simulink model "sampleModel1463"  (R2023a)
settings: Solver=VariableStepAuto  StartTime=0.0  StopTime=10.0  RelTol=1e-3
libraries: hdlsllib x2, simulink x1
settings Model: Creator=user1  LastModifiedBy=user1

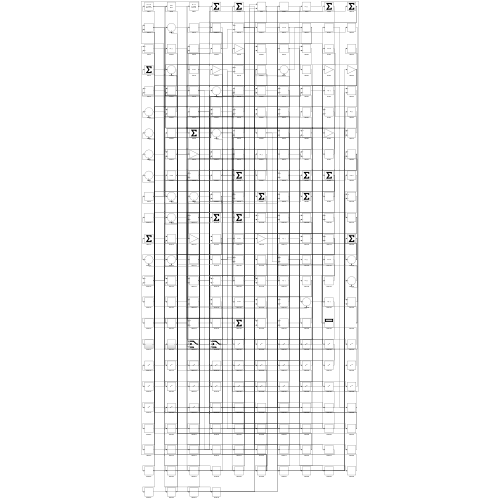
[thumbnail: Simulink's stored preview of the top-level diagram]
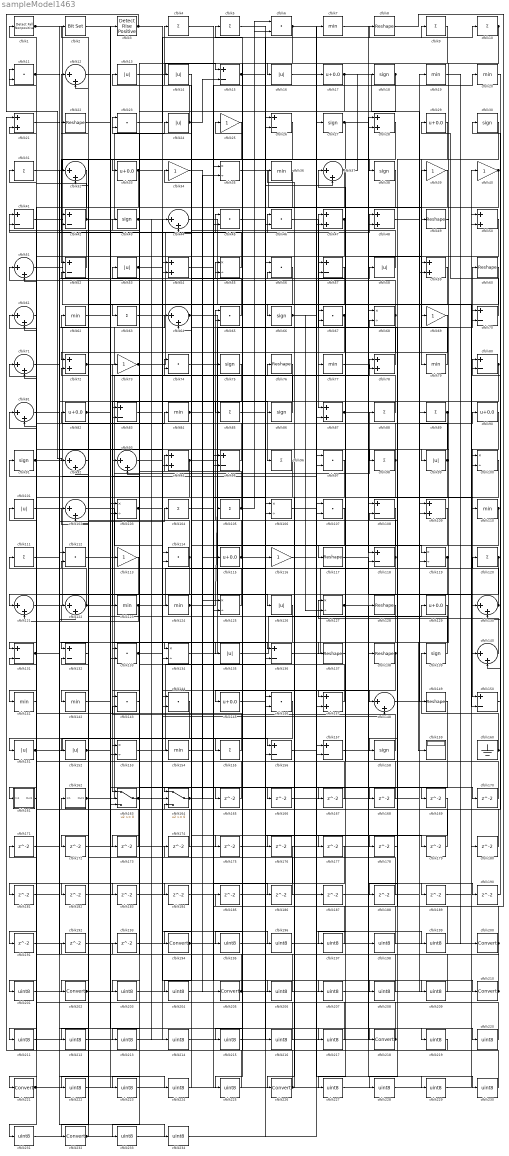
== system sampleModel1463 ==
  cfblk1 : hdlsllib/Logic and Bit Operations/Detect Fall Nonpositive  vinit=0  OutDataTypeStr=boolean
  cfblk{4..5,9..10,31,63,85,88..89,96,98,104..105,111,120,155} (16 alike) : Sum  Inputs=+
  cfblk{35,55,68,100,103,106,119,125,127,134,153} (11 alike) : Product  Inputs=*/  RndMeth=Zero  SaturateOnIntegerOverflow=on
  cfblk{13..14,16,24,53,58,99,101,126,135,151..152} (12 alike) : Abs  SaturateOnIntegerOverflow=off
  cfblk{12,32,37,44,51,61,64,71,81,92..93,102,121..122,130,140,148} (17 alike) : Sum  Inputs=|++
  cfblk{6,11,23,45..46,56,65,67,74,97,107,112,114,133,143..144,146} (17 alike) : DotProduct  OutDataTypeStr=Inherit: Inherit via internal rule
  cfblk{15,26,41..42,52,57,70,80,83,95,108,118,131..132,136,150,156..157} (18 alike) : Sum  Inputs=+-
  cfblk{21,28,47..48,50,54,59,72,78,87,94,109,147} (13 alike) : Sum
  cfblk{7,19..20,36,62,77,79,84,110,123..124,141..142,154} (14 alike) : MinMax
  cfblk{25,34,39..40,69,73,113,116} (8 alike) : Gain
  cfblk{17,29,33,82,90,115,129,145} (8 alike) : Bias  Bias=0.0  SaturateOnIntegerOverflow=off
  cfblk{8,22,49,60,76,117,128,137..138,149} (10 alike) : Reshape
  cfblk{18,27,30,38,43,66,75,86,91,139,158} (11 alike) : Signum
  cfblk159 : Display
  cfblk160 : Ground
  cfblk161 : Subsystem
      settings: LibrarySourceBlock=|
      | hdlsllib/Ports &
      | Subsystems/Subsystem
  cfblk162 : Subsystem
      settings: LibrarySourceBlock=|
      | hdlsllib/Ports &
      | Subsystems/Subsystem
  cfblk163 : Switch  SaturateOnIntegerOverflow=off  InputSameDT=off
  cfblk164 : Switch  SaturateOnIntegerOverflow=off  InputSameDT=off
  cfblk{165..193} (29 alike) : Delay  SampleTime=1
  cfblk{194,200,202,205,210,218,221,226,232} (9 alike) : DataTypeConversion  SaturateOnIntegerOverflow=off  RndMeth=Floor
  cfblk{195..199,201,203..204,206..209,211..217,219..220,222..225,227..231,233..234} (32 alike) : DataTypeConversion  OutDataTypeStr=uint8  SaturateOnIntegerOverflow=off  RndMeth=Floor
  cfblk2 : simulink/Logic and Bit Operations/Bit Set  iBit=0
      settings: LibrarySourceBlock=|
      | hdlsllib/Logic and Bit
      | Operations/Bit Set
  cfblk3 : hdlsllib/Logic and Bit Operations/Detect Rise Positive  vinit=0  OutDataTypeStr=boolean
  wires:
  cfblk58/1 -> cfblk23/1
  cfblk162/1(Out1) -> cfblk88/1, cfblk42/2
  cfblk122/1 -> cfblk76/1, cfblk112/2, cfblk61/2
  cfblk91/1 -> cfblk84/1, cfblk48/1
  cfblk114/1 -> cfblk62/1, cfblk141/1, cfblk121/1
  cfblk76/1 -> cfblk163/1
  cfblk115/1 -> cfblk65/1, cfblk209/1
  cfblk160/1 -> cfblk139/1, cfblk80/1
  cfblk138/1 -> cfblk165/1, cfblk166/1
  cfblk112/1 -> cfblk78/1
  cfblk152/1 -> cfblk55/2, cfblk219/1
  cfblk94/1 -> cfblk47/1, cfblk153/2, cfblk231/1
  cfblk1/1 -> cfblk118/1, cfblk94/2
  cfblk49/1 -> cfblk159/1
  cfblk107/1 -> cfblk194/1
  cfblk121/1 -> cfblk46/1
  cfblk70/1 -> cfblk29/1
  cfblk29/1 -> cfblk79/1
  cfblk79/1 -> cfblk39/1
  cfblk22/1 -> cfblk155/1
  cfblk87/1 -> cfblk147/1, cfblk110/1
  cfblk109/1 -> cfblk117/1
  cfblk128/1 -> cfblk133/1
  cfblk63/1 -> cfblk66/1
  cfblk134/1 -> cfblk60/1
  cfblk3/1 -> cfblk92/1, cfblk196/1
  cfblk45/1 -> cfblk8/1
  cfblk18/1 -> cfblk85/1, cfblk195/1
  cfblk151/1 -> cfblk156/1, cfblk55/1, cfblk131/2
  cfblk64/1 -> cfblk119/1, cfblk186/1
  cfblk62/1 -> cfblk3/1
  cfblk95/1 -> cfblk83/1
  cfblk126/1 -> cfblk143/1
  cfblk24/1 -> cfblk4/1, cfblk15/2
  cfblk98/1 -> cfblk57/2, cfblk175/1
  cfblk6/1 -> cfblk16/1, cfblk230/1
  cfblk90/1 -> cfblk150/1
  cfblk161/1(Out1) -> cfblk11/1
  cfblk74/1 -> cfblk126/1
  cfblk43/1 -> cfblk164/2, cfblk208/1
  cfblk9/1 -> cfblk145/1
  cfblk129/1 -> cfblk134/1
  cfblk44/1 -> cfblk87/1
  cfblk40/1 -> cfblk92/2, cfblk158/1, cfblk44/2
  cfblk99/1 -> cfblk113/1, cfblk72/2, cfblk61/1
  cfblk56/1 -> cfblk63/1
  cfblk135/1 -> cfblk129/1
  cfblk139/1 -> cfblk91/1
  cfblk20/1 -> cfblk162/1(In1)
  cfblk17/1 -> cfblk149/1, cfblk153/1
  cfblk27/1 -> cfblk70/2, cfblk167/1
  cfblk78/1 -> cfblk13/1
  cfblk19/1 -> cfblk200/1
  cfblk31/1 -> cfblk38/1
  cfblk35/1 -> cfblk49/1
  cfblk146/1 -> cfblk232/1
  cfblk13/1 -> cfblk15/1
  cfblk46/1 -> cfblk77/1
  cfblk15/1 -> cfblk119/2, cfblk6/1, cfblk69/1, cfblk178/1
  cfblk37/1 -> cfblk133/2, cfblk18/1
  cfblk21/1 -> cfblk218/1
  cfblk150/1 -> cfblk30/1
  cfblk60/1 -> cfblk72/1
  cfblk97/1 -> cfblk202/1
  cfblk88/1 -> cfblk53/1
  cfblk104/1 -> cfblk75/1
  cfblk33/1 -> cfblk114/2, cfblk163/3
  cfblk118/1 -> cfblk132/1, cfblk94/1
  cfblk148/1 -> cfblk90/1
  cfblk72/1 -> cfblk7/1, cfblk58/1
  cfblk32/1 -> cfblk131/1
  cfblk110/1 -> cfblk136/2, cfblk225/1
  cfblk53/1 -> cfblk134/2, cfblk148/1
  cfblk55/1 -> cfblk41/1
  cfblk54/1 -> cfblk210/1
  cfblk153/1 -> cfblk116/1
  cfblk123/1 -> cfblk46/2, cfblk121/2
  cfblk141/1 -> cfblk31/1
  cfblk136/1 -> cfblk68/1
  cfblk68/1 -> cfblk51/1, cfblk102/2
  cfblk131/1 -> cfblk104/1, cfblk136/1
  cfblk84/1 -> cfblk95/2, cfblk64/2, cfblk20/1
  cfblk52/1 -> cfblk12/1
  cfblk80/1 -> cfblk96/1, cfblk144/2, cfblk228/1
  cfblk106/1 -> cfblk10/1
  cfblk81/1 -> cfblk86/1
  cfblk2/1 -> cfblk156/2
  cfblk41/1 -> cfblk109/2
  cfblk10/1 -> cfblk99/1, cfblk33/1
  cfblk133/1 -> cfblk124/1, cfblk45/1
  cfblk113/1 -> cfblk152/1
  cfblk120/1 -> cfblk140/2, cfblk188/1
  cfblk158/1 -> cfblk143/2
  cfblk28/1 -> cfblk52/1
  cfblk119/1 -> cfblk142/1, cfblk176/1, cfblk177/1
  cfblk48/1 -> cfblk89/1
  cfblk124/1 -> cfblk105/1, cfblk125/1, cfblk115/1
  cfblk105/1 -> cfblk41/2, cfblk6/2
  cfblk89/1 -> cfblk151/1, cfblk161/1(In1)
  cfblk155/1 -> cfblk71/1
  cfblk4/1 -> cfblk106/2
  cfblk163/1 -> cfblk48/2, cfblk214/1
  cfblk65/1 -> cfblk14/1
  cfblk42/1 -> cfblk24/1, cfblk11/2
  cfblk66/1 -> cfblk127/2, cfblk199/1
  cfblk117/1 -> cfblk130/1
  cfblk103/1 -> cfblk154/1, cfblk148/2
  cfblk30/1 -> cfblk98/1
  cfblk83/1 -> cfblk135/1
  cfblk101/1 -> cfblk47/2
  cfblk73/1 -> cfblk56/2, cfblk223/1
  cfblk164/1 -> cfblk35/1, cfblk35/2
  cfblk11/1 -> cfblk125/2, cfblk234/1
  cfblk7/1 -> cfblk59/1
  cfblk77/1 -> cfblk78/2
  cfblk47/1 -> cfblk81/2, cfblk51/2
  cfblk127/1 -> cfblk189/1, cfblk190/1
  cfblk82/1 -> cfblk169/1, cfblk170/1
  cfblk71/1 -> cfblk64/1
  cfblk100/1 -> cfblk226/1
  cfblk145/1 -> cfblk37/2
  cfblk86/1 -> cfblk73/1
  cfblk61/1 -> cfblk71/2
  cfblk59/1 -> cfblk147/2
  cfblk51/1 -> cfblk150/2
  cfblk142/1 -> cfblk74/1
  cfblk125/1 -> cfblk74/2
  cfblk130/1 -> cfblk2/1, cfblk120/1, cfblk57/1
  cfblk102/1 -> cfblk144/1
  cfblk50/1 -> cfblk221/1
  cfblk12/1 -> cfblk67/1
  cfblk34/1 -> cfblk205/1
  cfblk23/1 -> cfblk9/1
  cfblk67/1 -> cfblk164/1, cfblk212/1
  cfblk69/1 -> cfblk137/1
  cfblk132/1 -> cfblk42/1
  cfblk147/1 -> cfblk43/1
  cfblk140/1 -> cfblk127/1
  cfblk156/1 -> cfblk17/1
  cfblk165/1 -> cfblk1/1
  cfblk166/1 -> cfblk59/2
  cfblk167/1 -> cfblk83/2
  cfblk39/1 -> cfblk168/1
  cfblk168/1 -> cfblk37/1
  cfblk170/1 -> cfblk67/2
  cfblk171/1 -> cfblk122/2
  cfblk92/1 -> cfblk172/1
  cfblk172/1 -> cfblk56/1
  cfblk143/1 -> cfblk173/1
  cfblk173/1 -> cfblk81/1
  cfblk174/1 -> cfblk52/2
  cfblk175/1 -> cfblk118/2
  cfblk178/1 -> cfblk68/2
  cfblk16/1 -> cfblk179/1
  cfblk179/1 -> cfblk103/1
  cfblk180/1 -> cfblk23/2
  cfblk144/1 -> cfblk181/1
  cfblk181/1 -> cfblk32/1
  cfblk25/1 -> cfblk182/1
  cfblk182/1 -> cfblk109/1
  cfblk36/1 -> cfblk183/1
  cfblk183/1 -> cfblk44/1
  cfblk14/1 -> cfblk184/1
  cfblk184/1 -> cfblk87/2
  cfblk8/1 -> cfblk185/1
  cfblk186/1 -> cfblk163/2
  cfblk116/1 -> cfblk187/1
  cfblk188/1 -> cfblk132/2
  cfblk189/1 -> cfblk140/1
  cfblk190/1 -> cfblk130/2
  cfblk96/1 -> cfblk191/1
  cfblk191/1 -> cfblk106/1
  cfblk192/1 -> cfblk28/1
  cfblk193/1 -> cfblk114/1
  cfblk194/1 -> cfblk80/2, cfblk128/1
  cfblk195/1 -> cfblk107/1
  cfblk196/1 -> cfblk107/2
  cfblk108/1 -> cfblk197/1
  cfblk197/1 -> cfblk95/1
  cfblk187/1 -> cfblk198/1
  cfblk198/1 -> cfblk108/1
  cfblk199/1 -> cfblk108/2
  cfblk200/1 -> cfblk193/1, cfblk70/1
  cfblk38/1 -> cfblk201/1
  cfblk201/1 -> cfblk19/1
  cfblk202/1 -> cfblk103/2, cfblk82/1
  cfblk75/1 -> cfblk203/1
  cfblk203/1 -> cfblk97/1
  cfblk169/1 -> cfblk204/1
  cfblk204/1 -> cfblk97/2
  cfblk205/1 -> cfblk171/1, cfblk22/1, cfblk40/1
  cfblk154/1 -> cfblk206/1
  cfblk206/1 -> cfblk34/1
  cfblk93/1 -> cfblk207/1
  cfblk207/1 -> cfblk138/1
  cfblk208/1 -> cfblk93/1
  cfblk209/1 -> cfblk93/2
  cfblk210/1 -> cfblk112/1, cfblk101/1
  cfblk176/1 -> cfblk211/1
  cfblk211/1 -> cfblk54/1
  cfblk212/1 -> cfblk54/2
  cfblk26/1 -> cfblk213/1
  cfblk213/1 -> cfblk28/2
  cfblk214/1 -> cfblk26/1
  cfblk177/1 -> cfblk215/1
  cfblk215/1 -> cfblk26/2
  cfblk5/1 -> cfblk216/1
  cfblk216/1 -> cfblk192/1
  cfblk85/1 -> cfblk217/1
  cfblk217/1 -> cfblk5/1
  cfblk218/1 -> cfblk12/2, cfblk122/1
  cfblk219/1 -> cfblk21/1
  cfblk185/1 -> cfblk220/1
  cfblk220/1 -> cfblk21/2
  cfblk221/1 -> cfblk45/2, cfblk123/1
  cfblk57/1 -> cfblk222/1
  cfblk222/1 -> cfblk50/1
  cfblk223/1 -> cfblk50/2
  cfblk111/1 -> cfblk224/1
  cfblk224/1 -> cfblk174/1
  cfblk225/1 -> cfblk111/1
  cfblk226/1 -> cfblk164/3, cfblk65/2, cfblk36/1, cfblk25/1, cfblk102/1
  cfblk137/1 -> cfblk227/1
  cfblk227/1 -> cfblk100/1
  cfblk228/1 -> cfblk100/2
  cfblk157/1 -> cfblk229/1
  cfblk229/1 -> cfblk180/1
  cfblk230/1 -> cfblk157/1
  cfblk231/1 -> cfblk157/2
  cfblk232/1 -> cfblk32/2, cfblk27/1
  cfblk149/1 -> cfblk233/1
  cfblk233/1 -> cfblk146/1
  cfblk234/1 -> cfblk146/2

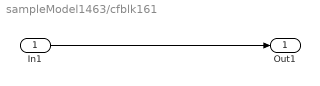
== system sampleModel1463/cfblk161 ==
  In1 : Inport
  Out1 : Outport
  wires:
  In1/1 -> Out1/1

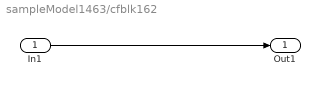
== system sampleModel1463/cfblk162 ==
  In1 : Inport
  Out1 : Outport
  wires:
  In1/1 -> Out1/1
